simulink model "mVarBus_ref"
settings: Solver=FixedStepDiscrete  StartTime=0.0  StopTime=10.0  RelTol=1e-3
PreLoadFcn:
  | load mvardims_bus3.mat;
settings Model: ExtModeAutoUpdateStatusClock=off  Creator=djia  LastModifiedBy=hungdang
settings DataIOCC: LimitDataPoints=on  SaveFormat=Structure  SignalLoggingSaveFormat=ModelDataLogs  ReturnWorkspaceOutputs=off
settings OptimizationCC: InlineParams=on  ExpressionDepthLimit=2147483647  InitFltsAndDblsToZero=on  EfficientMapNaN2IntZero=off  OptimizeModelRefInitCode=on  LifeSpan=1  SimCompilerOptimization=Off
settings DebuggingCC: ReadBeforeWriteMsg=DisableAll  WriteAfterWriteMsg=DisableAll  WriteAfterReadMsg=DisableAll  UnderspecifiedInitializationDetection=Classic  MergeDetectMultiDrivingBlocksExec=none  SignalResolutionControl=TryResolveAllWithWarning  SolverPrmCheckMsg=warning  FcnCallInpInsideContextMsg=UseLocalSettings  FrameProcessingCompatibilityMsg=warning  ModelReferenceSymbolNameMessage=none  StateNameClashWarn=warning  SFUnexpectedBacktrackingDiag=warning  SFNoUnconditionalDefaultTransitionDiag=warning
settings HardwareCC: ProdBitPerPointer=32  ProdLargestAtomicFloat=None  ProdIntDivRoundTo=Undefined  ProdEndianess=Unspecified  ProdWordSize=32  ProdHWDeviceType=32-bit Generic
settings ModelReferenceCC: PropagateSignalLabelsOutOfModel=off
settings SFSimCC: SimUseLocalCustomCode=off
settings RTWCC: SystemTargetFile=ert.tlc  TemplateMakefile=ert_default_tmf  Description=Real-Time Workshop Embedded Coder (no auto configuration)  RetainRTWFile=on  ProcessScript=ert_make_rtw_hook  RTWUseLocalCustomCode=off  RTWCompilerOptimization=Off
settings CodeAppCC: IgnoreCustomStorageClasses=off  MaxIdLength=63  CustomSymbolStrType=$N$R$M  InternalIdentifier=Classic
settings ERTTargetCC: CodeReplacementLibrary=ANSI_C  MultiwordLength=2048  GenerateSampleERTMain=on  MatFileLogging=on  InlinedParameterPlacement=NonHierarchical  ERTCustomFileTemplate=example_file_process.tlc  ConvertIfToSwitch=off  SuppressUnreachableDefaultCases=off

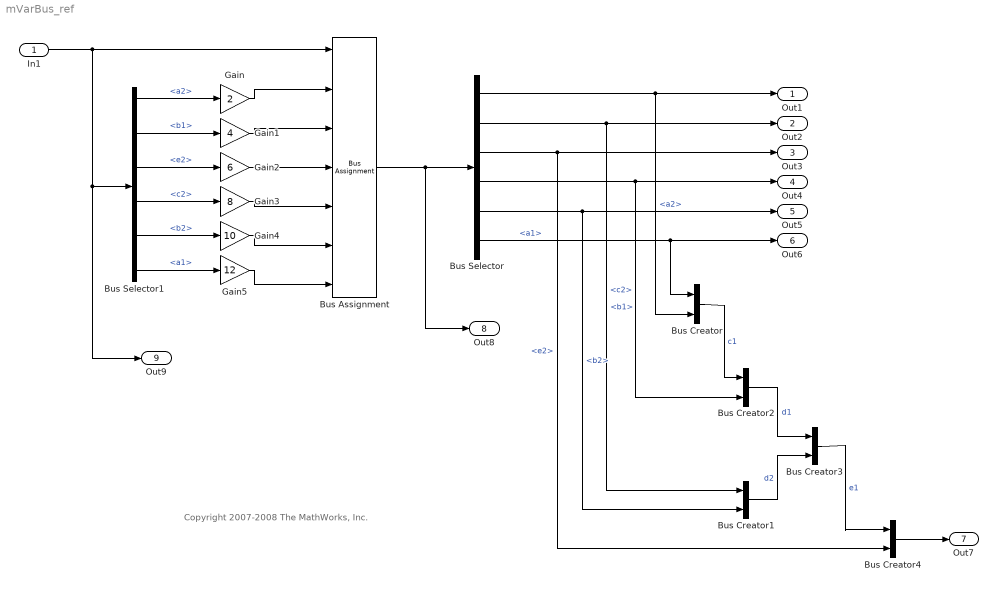
== system mVarBus_ref ==
  note: Copyright 2007-2008 The MathWorks, Inc.
  In1 : Inport  OutDataTypeStr=Bus: e  Interpolate=off  BusOutputAsStruct=on
  Bus Assignment : BusAssignment  AssignedSignals=e1.d1.c1.a2,e1.d2.b1,e2,e1.d1.c2,e1.d2.b2,e1.d1.c1.a1
  Bus Creator : BusCreator  Inputs=2  OutDataTypeStr=Bus: a  NonVirtualBus=on
  Bus Creator1 : BusCreator  Inputs=2  OutDataTypeStr=Bus: b  NonVirtualBus=on
  Bus Creator2 : BusCreator  Inputs=2  OutDataTypeStr=Bus: c  NonVirtualBus=on
  Bus Creator3 : BusCreator  Inputs=2  OutDataTypeStr=Bus: d  NonVirtualBus=on
  Bus Creator4 : BusCreator  Inputs=2  OutDataTypeStr=Bus: e  NonVirtualBus=on
  Bus Selector : BusSelector  OutputSignals=e1.d1.c1.a2,e1.d2.b1,e2,e1.d1.c2,e1.d2.b2,e1.d1.c1.a1
  Bus Selector1 : BusSelector  OutputSignals=e1.d1.c1.a2,e1.d2.b1,e2,e1.d1.c2,e1.d2.b2,e1.d1.c1.a1
  Gain : Gain  Gain=2
  Gain1 : Gain  Gain=4
  Gain2 : Gain  Gain=6
  Gain3 : Gain  Gain=8
  Gain4 : Gain  Gain=10
  Gain5 : Gain  Gain=12
  Out1 : Outport
  Out2 : Outport  Port=2
  Out3 : Outport  Port=3
  Out4 : Outport  Port=4
  Out5 : Outport  Port=5
  Out6 : Outport  Port=6
  Out7 : Outport  Port=7  OutDataTypeStr=Bus: e  BusOutputAsStruct=on
  Out8 : Outport  Port=8  OutDataTypeStr=Bus: e  BusOutputAsStruct=on
  Out9 : Outport  Port=9  OutDataTypeStr=Bus: e  BusOutputAsStruct=on
  wires:
  Bus Selector/1 -> Out1/1, Bus Creator/2  "<a2>"
  Bus Selector/2 -> Out2/1, Bus Creator1/1  "<b1>"
  Bus Selector/3 -> Out3/1, Bus Creator4/2  "<e2>"
  Bus Selector/4 -> Out4/1, Bus Creator2/2  "<c2>"
  Bus Selector/5 -> Out5/1, Bus Creator1/2  "<b2>"
  Bus Selector/6 -> Out6/1, Bus Creator/1  "<a1>"
  In1/1 -> Bus Assignment/1, Bus Selector1/1, Out9/1
  Bus Selector1/1 -> Gain/1  "<a2>"
  Bus Selector1/2 -> Gain1/1  "<b1>"
  Bus Selector1/3 -> Gain2/1  "<e2>"
  Bus Selector1/4 -> Gain3/1  "<c2>"
  Bus Selector1/5 -> Gain4/1  "<b2>"
  Bus Selector1/6 -> Gain5/1  "<a1>"
  Bus Assignment/1 -> Bus Selector/1, Out8/1
  Gain/1 -> Bus Assignment/2
  Gain1/1 -> Bus Assignment/3
  Gain2/1 -> Bus Assignment/4
  Gain3/1 -> Bus Assignment/5
  Gain4/1 -> Bus Assignment/6
  Gain5/1 -> Bus Assignment/7
  Bus Creator/1 -> Bus Creator2/1  "c1"
  Bus Creator2/1 -> Bus Creator3/1  "d1"
  Bus Creator1/1 -> Bus Creator3/2  "d2"
  Bus Creator3/1 -> Bus Creator4/1  "e1"
  Bus Creator4/1 -> Out7/1
